simulink model "tweede_orde_allpass"  (Simulink 6.6)
settings: Solver=ode45  StartTime=0.0  StopTime=inf  RelTol=1e-3
libraries: simulink x2, dspsrcs4 x1, simulink_extras x1
settings Model: Creator=student  LastModifiedBy=student

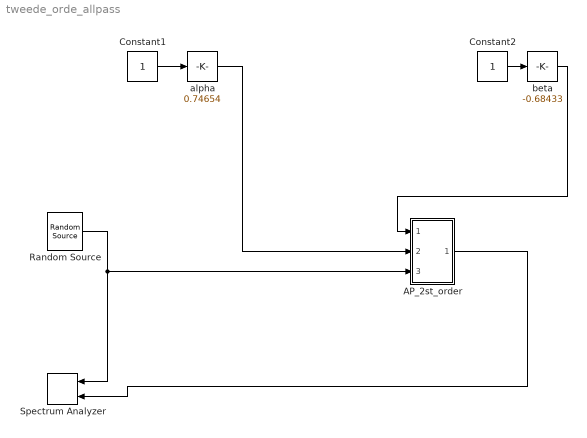
== system tweede_orde_allpass ==
  AP_2st_order : Subsystem
  Constant1 : Constant
  Constant2 : Constant
  Random Source : dspsrcs4/Random Source  SrcType=Uniform  NormMethod=Ziggurat  CltLength=12  MinVal=-10  MaxVal=10  MeanVal=0  VarVal=1  RepMode=Not repeatable  rawSeed=1  IsInherit=off  SampMode=Discrete  SampTime=1  SampFrame=1  DataType=Double  OutComplex=Real
  Spectrum Analyzer : simulink_extras/Additional Sinks/Spectrum Analyzer  Orientation=left  SystemSampleTime=-1  npts=1024  fftpts=1024  HowOften=64  sampleT=1
  alpha : simulink/Math Operations/Slider Gain  SystemSampleTime=-1  low=0  gain=0.74654  high=0.9
  beta : simulink/Math Operations/Slider Gain  SystemSampleTime=-1  low=-0.9  gain=-0.68433  high=0.9
  wires:
  alpha/1 -> AP_2st_order/2(alfa)
  Constant1/1 -> alpha/1
  Random Source/1 -> Spectrum Analyzer/1, AP_2st_order/3(source)
  beta/1 -> AP_2st_order/1(beta)
  Constant2/1 -> beta/1
  AP_2st_order/1(Out1) -> Spectrum Analyzer/2

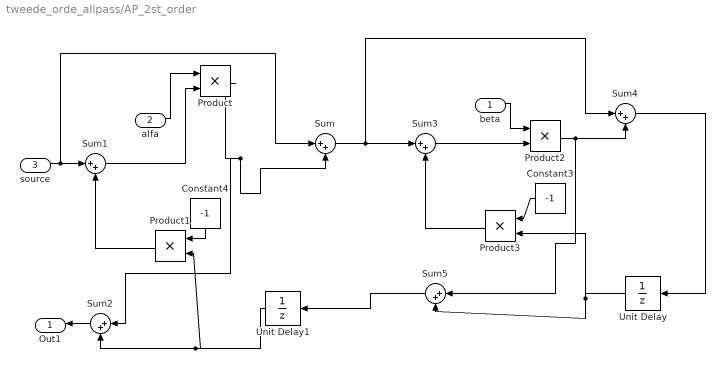
== system tweede_orde_allpass/AP_2st_order ==
  beta : Inport
  alfa : Inport  Port=2
  source : Inport  Port=3
  Constant3 : Constant  Orientation=left  Value=-1
  Constant4 : Constant  Orientation=down  Value=-1
  Product : Product  RndMeth=Zero
  Product1 : Product  Orientation=left  RndMeth=Zero
  Product2 : Product  RndMeth=Zero
  Product3 : Product  Orientation=left  RndMeth=Zero
  Sum{,1,3..4} (4 alike) : Sum  Inputs=|++
  Sum2 : Sum  Orientation=left  Inputs=|++
  Sum5 : Sum  Orientation=left  Inputs=|++
  Unit Delay : UnitDelay  Orientation=left
  Unit Delay1 : UnitDelay  Orientation=left
  Out1 : Outport  Orientation=left
  wires:
  Sum1/1 -> Product/2
  Product1/1 -> Sum1/2
  Product/1 -> Sum/2, Sum2/1
  Sum/1 -> Sum3/1, Sum4/1
  Sum3/1 -> Product2/2
  Product2/1 -> Sum4/2, Sum5/1
  Sum4/1 -> Unit Delay/1
  Unit Delay/1 -> Sum5/2, Product3/2
  Product3/1 -> Sum3/2
  Constant3/1 -> Product3/1
  Sum5/1 -> Unit Delay1/1
  Unit Delay1/1 -> Sum2/2, Product1/2
  Constant4/1 -> Product1/1
  source/1 -> Sum1/1, Sum/1
  beta/1 -> Product2/1
  alfa/1 -> Product/1
  Sum2/1 -> Out1/1
